simulink model "rl_watertank"  (R2023a)
settings: Solver=VariableStepAuto  StartTime=0.0  StopTime=300  RelTol=1e-3
values from neighbouring files (symbols this model uses):
  A1 = 0.0154    [parametros.m]    (also in variables.mat)
  A2 = 5e-5    (= 5e-05)    [parametros.m]    (also in variables.mat)
  az = 0.5    [parametros.m]    (also in variables.mat)
  g = 9.8    [parametros.m]    (also in variables.mat)
  H_star = H_max/2    (= 0.31)    [parametros.m]    (also in variables.mat)
  Q_star = ro*A2*az*sqrt(2*g*H_star)    [parametros.m]    (also in variables.mat = 0.0616238590158)
  Qmax = 0.1    [parametros.m]    (also in variables.mat)
  ro = 1000    [parametros.m]    (also in variables.mat)
libraries: rllib x1
settings Model: Creator=emmanuel  LastModifiedBy=empg0
settings OptimizationCC: ReuseModelBlockBuffer=off

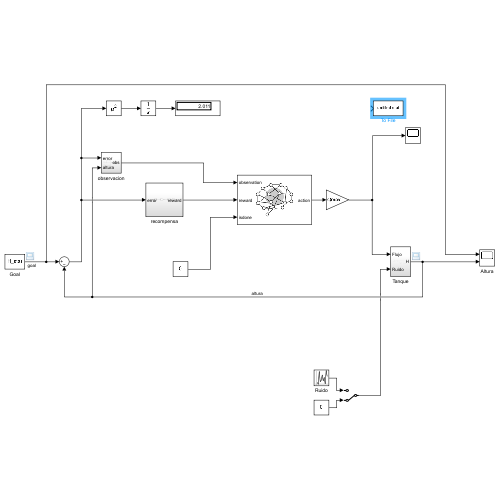
[thumbnail: Simulink's stored preview of the top-level diagram]
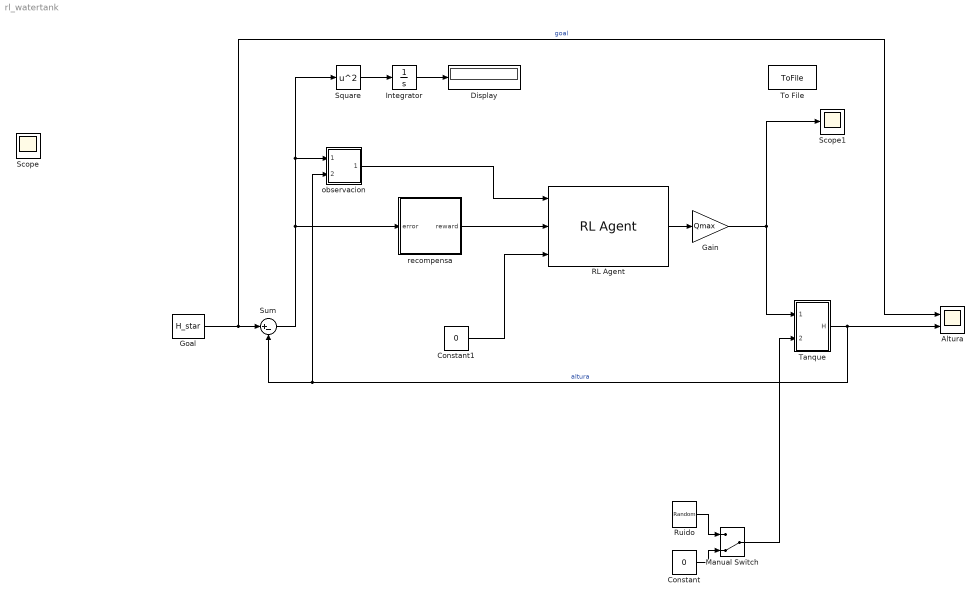
== system rl_watertank ==
  Altura : Scope  NumInputPorts=2
  Constant : Constant  Value=0
  Constant1 : Constant  Value=0
  Display : Display
  Gain : Gain  Gain=Qmax
  Goal : Constant  Value=H_star
  Integrator : Integrator
  Manual Switch : ManualSwitch  CurrentSetting=0
  RL Agent : rllib/RL Agent  Agent=agent  ExternalActionAsInput=off  ProvideLastAction=off  ProvideCumRwd=off  TreatAsDirectFeedthrough=on  UseStrictObservationDataTypes=off
  Ruido : UniformRandomNumber  Minimum=-Q_star*0.2  Maximum=Q_star*0.2  Seed=140  SampleTime=0.5
  Scope1 : Scope
  Square : Math  Operator=square  SignedPower=on  RndMeth=Zero
  Sum : Sum  Inputs=|+-
  Tanque : Subsystem
  To File : ToFile  SaveFormat=Timeseries
  observacion : Subsystem
  recompensa : Subsystem
  Scope : Scope
  wires:
  Tanque/1(H) -> Altura/2, observacion/2(altura), Sum/2  "altura"
  Ruido/1 -> Manual Switch/1
  Constant/1 -> Manual Switch/2
  Manual Switch/1 -> Tanque/2(Ruido)
  Sum/1 -> observacion/1(error), Square/1, recompensa/1(error)
  observacion/1(obs) -> RL Agent/1
  Goal/1 -> Altura/1, Sum/1  "goal"
  Constant1/1 -> RL Agent/3
  recompensa/1(reward) -> RL Agent/2
  Square/1 -> Integrator/1
  Integrator/1 -> Display/1
  RL Agent/1 -> Gain/1
  Gain/1 -> Tanque/1(Flujo), Scope1/1

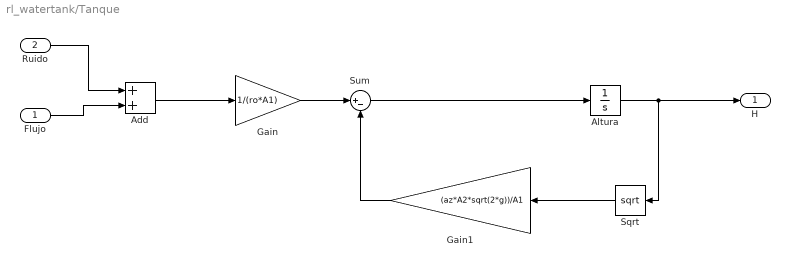
== system rl_watertank/Tanque ==
  Flujo : Inport
  Ruido : Inport  Port=2
  Add : Sum
  Altura : Integrator  LimitOutput=on  UpperSaturationLimit=0.62  LowerSaturationLimit=0
  Gain : Gain  Gain=1/(ro*A1)
  Gain1 : Gain  Gain=(az*A2*sqrt(2*g))/A1
  Sqrt : Sqrt
  Sum : Sum  Inputs=|+-
  H : Outport
  wires:
  Gain/1 -> Sum/1
  Sum/1 -> Altura/1
  Sqrt/1 -> Gain1/1
  Gain1/1 -> Sum/2
  Altura/1 -> H/1, Sqrt/1
  Add/1 -> Gain/1
  Flujo/1 -> Add/2
  Ruido/1 -> Add/1

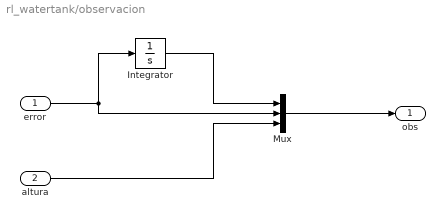
== system rl_watertank/observacion ==
  error : Inport
  altura : Inport  Port=2
  Integrator : Integrator
  Mux : Mux  Inputs=3
  obs : Outport
  wires:
  Integrator/1 -> Mux/1
  error/1 -> Integrator/1, Mux/2
  Mux/1 -> obs/1
  altura/1 -> Mux/3

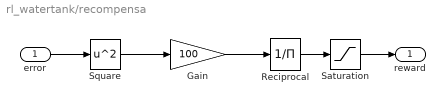
== system rl_watertank/recompensa ==
  error : Inport
  Gain : Gain  Gain=100
  Reciprocal : Product  Inputs=/  RndMeth=Zero  SaturateOnIntegerOverflow=on
  Saturation : Saturate  UpperLimit=100  LowerLimit=0
  Square : Math  Operator=square
  reward : Outport
  wires:
  error/1 -> Square/1
  Gain/1 -> Reciprocal/1
  Square/1 -> Gain/1
  Reciprocal/1 -> Saturation/1
  Saturation/1 -> reward/1
